simulink model "MavicProComplete"  (R2019a)
settings: Solver=VariableStepAuto  StartTime=0  StopTime=250  FixedStep=.01  MaxStep=10  MinStep=.001  RelTol=1e-4  EnableMultiTasking=on
InitFcn:
  | addpath params;
  | addpath fcns;
  | load batteryParams;
  | load motorParams;
  | load ukfBatteryParams;
  | load DJI.mat;
  | load DJIquadModel_X.mat;
model workspace (MAT data in the model file):
  Sig = Simulink.Signal
  Sig.DataType = 'auto'
  Sig.Dimensions = -1
  Sig.DimensionsMode = 'auto'
  Sig.Complexity = 'auto'
  Sig.SampleTime = -1
  Sig.SamplingMode = 'auto'
undefined symbols (not defined in the file): motorRes, P, Phi, Psi, Q, quadModel, R, The, Z
libraries: simulink x7, dspstat3 x5
(part 1 of 2)
Description:
  | This is a configurable quadcopter simulation.
  | This Simulink model demonstates attitude control.
  | 
  | Additional quadcopter modeling and simulation materials available at:
  | github.com/dch33/Quad-Sim
  | 
  | Copyright (C) 2014 D. Hartman, K. Landis, S. Moreno, J. Kim, M. Mehrer
  | 
  | License:
  |     This program is free software: you can redistribute it and/or modify
  |     it under the terms of the GNU LESSER GENERAL PUBLIC LICENSE as published by
  |     the Free Software Foundation, either version 3 of the License, or
  |     (at your option) any later version.
  | 
  |     This program is distributed in the hope that it will be useful,
  |     but WITHOUT ANY WARRANTY; without even the implied warranty of
  |     MERCHANTABILITY or FITNESS FOR A PARTICULAR PURPOSE.  See the
  |     GNU General Public License for more details.
  | 
  |     You should have received a copy of the GNU LESSER GENERAL PUBLIC LICENSE
  |     along with this program.  If not, see <http://www.gnu.org/licenses/>.
settings Model: ModifiedComment=tdarrah -- Tue Jun 04 09:34:35 2019 -- Version 1.40  Creator=David Hartman  LastModifiedBy=tdarrah
settings Model: ModifiedHistory=|
  | tdarrah -- Tue Jun 04 09:34:35 2019 -- Version 1.40
  | 
  | tdarrah -- Tue Jun 04 05:29:55 2019 -- Version 1.39
  | 
  | tdarrah -- Mon Jun 03 18:31:35 2019 -- Version 1.38
  | closed the battery loop
  | 
  | tdarrah -- Mon Jun 03 18:20:30 2019 -- Version 1.37
  | added battery
  | 
  | 
  | tdarrah -- Mon Jun 03 17:58:08 2019 -- Version 1.36
  | incorporated our motors in model
  | 
  | 
  | Sahai Couso -- Fri May 10 11:35:12 2019 -- Version 1.35
  | 
  | Sahai Couso -- Fri May 10 10:41:34 2019 -- Version 1.34
  | 
  | Sahai Couso -- Fri May 10 10:40:52 2019 -- Version 1.33
  | 
  | Sahai Couso -- Fri May 10 10:30:50 2019 -- Version 1.32
  | 
  | Sahai Couso -- Fri May 10 10:24:25 2019 -- Version 1.31
  | 
  | Sahai Couso -- Wed May 08 22:16:35 2019 -- Version 1.30
  | 
  | Sahai Couso -- Wed May 08 22:15:23 2019 -- Version 1.29
  | 
  | Sahai Couso -- Wed May 08 22:14:58 2019 -- Version 1.28
  | 
  | Sahai Couso -- Wed May 08 22:04:36 2019 -- Version 1.27
  | 
  | Sahai Couso -- Wed May 08 22:04:16 2019 -- Version 1.26
  | 
  | Sahai Couso -- Wed May 08 21:57:14 2019 -- Version 1.25
  | 
  | Sahai Couso -- Wed May 08 21:54:04 2019 -- Version 1.24
  | 
  | Sahai Couso -- Wed May 08 21:53:17 2019 -- Version 1.23
  | 
  | Sahai Couso -- Wed May 08 21:48:07 2019 -- Version 1.22
  | 
  | Sahai Couso -- Wed May 08 21:35:53 2019 -- Version 1.21
  | 
  | Sahai Couso -- Wed May 08 21:28:21 2019 -- Version 1.19
  | 
  | Sahai Couso -- Wed May 08 21:28:21 2019 -- Version 1.19
  | 
  | Sahai Couso -- Wed May 08 21:25:30 2019 -- Version 1.18
  | 
  | Sahai Couso -- Wed May 08 21:23:06 2019 -- Version 1.17
  | 
  | Sahai Couso -- Wed May 08 13:57:34 2019 -- Version 1.16
  | 
  | Sahai Couso -- Wed May 08 00:58:43 2019 -- Version 1.15
  | 
  | Sahai Couso -- Wed May 08 00:58:03 2019 -- Version 1.14
  | 
  | Sahai Couso -- Tue May 07 23:55:58 2019 -- Version 1.13
  | 
  | Sahai Couso -- Tue May 07 23:08:00 2019 -- Version 1.12
  | 
  | Sahai Couso -- Tue May 07 23:06:52 2019 -- Version 1.11
  | 
  | Sahai Couso -- Tue May 07 22:57:09 2019 -- Version 1.10
  | 
  | Sahai Couso -- Tue May 07 22:48:57 2019 -- Version 1.9
  | 
  | Sahai Couso -- Tue May 07 21:40:08 2019 -- Version 1.8
  | 
  | Yves -- Tue Apr 04 13:12:37 2017 -- Version 1.7
  | 
  | Yves -- Tue Apr 04 13:10:33 2017 -- Version 1.6
  | 
  | davidhartman -- Fri Jun 06 23:19:51 2014 -- Version 1.5
  | 
  | 
  | davidhartman -- Fri Jun 06 22:53:10 2014 -- Version 1.3
settings SolverCC: AlgebraicLoopSolver=LineSearch  AutoInsertRateTranBlk=on
settings DataIOCC: SaveFormat=Array  SignalLogging=off  ReturnWorkspaceOutputs=off
settings OptimizationCC: DefaultParameterBehavior=Inlined  LifeSpan=inf
settings DebuggingCC: UnderspecifiedInitializationDetection=Classic  MergeDetectMultiDrivingBlocksExec=none  SolverPrmCheckMsg=warning  UniqueDataStoreMsg=warning  StateNameClashWarn=warning  StrictBusMsg=WarnOnBusTreatedAsVector  SFUnexpectedBacktrackingDiag=warning  SFNoUnconditionalDefaultTransitionDiag=warning  SFExecutionAtInitializationDiag=none  ArithmeticOperatorsInVariantConditions=warning
settings HardwareCC: ProdBitPerPointer=32  ProdBitPerSizeT=32  ProdBitPerPtrDiffT=32  ProdLargestAtomicFloat=None  ProdIntDivRoundTo=Undefined  ProdEndianess=Unspecified  ProdWordSize=32  ProdHWDeviceType=32-bit Generic
settings ModelReferenceCC: PropagateSignalLabelsOutOfModel=off
settings SFSimCC: SimUseLocalCustomCode=off
settings RTWCC: RTWUseLocalCustomCode=off
settings CodeAppCC: StateflowObjectComments=on
settings GRTTargetCC: TargetLangStandard=C89/C90 (ANSI)  GeneratePreprocessorConditionals=Disable all
settings ConfigComp: CovMetricSettings=dw  CovHtmlReporting=on  CovSaveCumulativeToWorkspaceVar=on  CovSaveSingleToWorkspaceVar=on  CovExternalEMLEnable=off

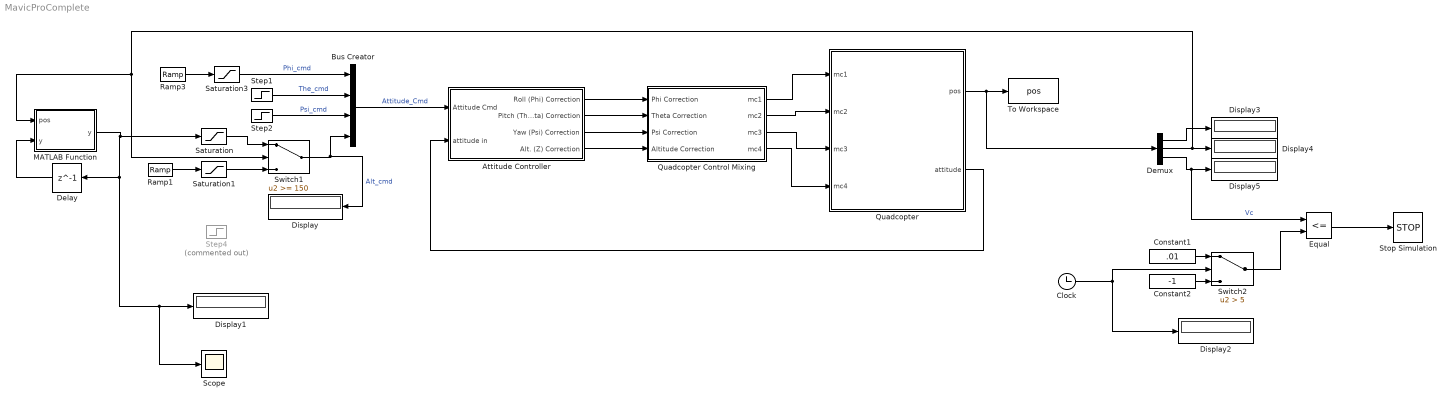
== system MavicProComplete ==
  Attitude Controller : Subsystem
  Bus Creator : BusCreator  Inputs=4
  Clock : Clock
  Constant1 : Constant  Value=.01
  Constant2 : Constant  Value=-1
  Delay : Delay  DelayLength=1  InitialCondition=10
  Demux : Demux  Outputs=3
  Display{,1..5} (6 alike) : Display
  Equal : RelationalOperator  Operator=<=  OutDataTypeStr=boolean  RndMeth=Simplest
  MATLAB Function : MATLAB Function  TreatAsAtomicUnit=on  SystemSampleTime=.1
      settings: MinAlgLoopOccurrences=on
  Quadcopter : Subsystem
  Quadcopter Control Mixing : Subsystem
  Ramp1 : simulink/Sources/Ramp  slope=.1  start=0  InitialOutput=0
  Ramp3 : simulink/Sources/Ramp  slope=-.0001  start=0  InitialOutput=0
  Saturation : Saturate  UpperLimit=10  LowerLimit=-1
  Saturation1 : Saturate  UpperLimit=10  LowerLimit=0
  Saturation3 : Saturate  UpperLimit=.002  LowerLimit=-.002
  Scope : Scope
  Step1 : Step  Time=1000000  After=10*pi/180  SampleTime=1
  Step2 : Step  Time=1000000  After=45*pi/180  SampleTime=1
  Step4 : Step  Commented=on  Time=0  Before=10  After=10  SampleTime=0
  Stop Simulation : Stop
  Switch1 : Switch  Threshold=150
  Switch2 : Switch  Criteria=u2 > Threshold  Threshold=5
  To Workspace : ToWorkspace  VariableName=pos  SampleTime=-1
      settings: Save2DSignal=2-D array (concatenate along first dimension)
  wires:
  Quadcopter/2(attitude) -> Attitude Controller/2(attitude in)
  Quadcopter Control Mixing/1(mc1) -> Quadcopter/1(mc1)
  Quadcopter Control Mixing/2(mc2) -> Quadcopter/2(mc2)
  Quadcopter Control Mixing/3(mc3) -> Quadcopter/3(mc3)
  Quadcopter Control Mixing/4(mc4) -> Quadcopter/4(mc4)
  Attitude Controller/1(Roll (Phi) Correction) -> Quadcopter Control Mixing/1(Phi Correction)
  Attitude Controller/2(Pitch (Theta) Correction) -> Quadcopter Control Mixing/2(Theta Correction)
  Attitude Controller/3(Yaw (Psi) Correction) -> Quadcopter Control Mixing/3(Psi Correction)
  Attitude Controller/4(Alt. (Z) Correction) -> Quadcopter Control Mixing/4(Altitude Correction)
  Saturation/1 -> Switch1/1
  Saturation3/1 -> Bus Creator/1  "Phi_cmd"
  Bus Creator/1 -> Attitude Controller/1(Attitude Cmd)  "Attitude_Cmd"
  Step2/1 -> Bus Creator/3  "Psi_cmd"
  Step1/1 -> Bus Creator/2  "The_cmd"
  Quadcopter/1(pos) -> Demux/1, To Workspace/1
  Saturation1/1 -> Switch1/3
  Ramp1/1 -> Saturation1/1
  Switch1/1 -> Display/1, Bus Creator/4  "Alt_cmd"
  Ramp3/1 -> Saturation3/1
  Demux/1 -> Display3/1
  Demux/2 -> MATLAB Function/1(pos), Switch1/2, Display4/1
  Demux/3 -> Equal/1, Display5/1  "Vc"
  Equal/1 -> Stop Simulation/1
  Constant1/1 -> Switch2/1
  Constant2/1 -> Switch2/3
  Switch2/1 -> Equal/2
  Clock/1 -> Switch2/2, Display2/1
  MATLAB Function/1(y) -> Scope/1, Display1/1, Delay/1, Saturation/1
  Delay/1 -> MATLAB Function/2("y ")

== system MavicProComplete/Attitude Controller ==
  Attitude Cmd : Inport
  attitude in : Inport  Port=2
  Altitude (Z) Control : Subsystem  mask{Kpz=3.0, Kiz=4.5, Kdz=3.0, LimitOutput=on, USat=1, LSat=-1, GOffset=(sqrt((quadModel.mass*quadModel.g)/(4*quadModel.ct))-quadModel.b)/quadModel.cr}
      mask prompts: Kpz "Kp"; Kiz "Ki"; Kdz "Kd"; LimitOutput "Integral Saturation?"; USat "Upper saturation limit:"; LSat "Lower saturation limit:"; GOffset "Gravity Feedforward"
      mask help:
      | Adjust PID controller gains through this mask interface, or "look under mask" for more detailed adjustments.
      |
      | Note: Gravity Offset will not appear on block face as a value until simulation is run if it is the result of a formula involving the quadcopter model parameters.
      mask TypeOptions Kpz: Kpz/Gain
      mask TypeOptions Kiz: Kiz/Gain
      mask TypeOptions Kdz: Kdz/Gain
      mask TypeOptions LimitOutput:
      | Integrator
      | Limited/LimitOutput
      mask TypeOptions USat:
      | Integrator
      | Limited/UpperSaturationLimit
      mask TypeOptions LSat:
      | Integrator
      | Limited/LowerSaturationLimit
      mask TypeOptions GOffset: Gravity Offset (Level Flight)/Value
      mask Display:
      | fprintf(['Gravity Offset = ' num2str(GOffset) '\n' ...
      |     'Kp = ' num2str(Kpz) '\n' ...
      |     'Ki = ' num2str(Kiz) '\n' ...
      |     'Kd = ' num2str(Kdz) '\n' ...
      |     'Integral Saturation: ' LimitOutput]);
      | if strcmp(LimitOutput,'on')
      |     fprintf([' \n' ' \n' ' \n' ' \n' ' \n' '\n' ...
      |         'Limits: ' num2str(USat) ' to ' num2str(LSat)]);
      | end
  Bus Selector : BusSelector  OutputSignals=Phi,P,The,Q,Psi,R,Z
  Pitch (Theta) Control : Subsystem  mask{Kpt=2, Kit=1.1, Kdt=1.2, LimitOutput=on, USat=1, LSat=-1}
      mask prompts: Kpt "Kp"; Kit "Ki"; Kdt "Kd"; LimitOutput "Integral Saturation?"; USat "Upper saturation limit:"; LSat "Lower saturation limit:"
      mask help: Adjust PID controller gains through this mask interface, or "look under mask" for more detailed adjustments.
      mask TypeOptions Kpt: Kpt/Gain
      mask TypeOptions Kit: Kit/Gain
      mask TypeOptions Kdt: Kdt/Gain
      mask TypeOptions LimitOutput:
      | Integrator
      | Limited/LimitOutput
      mask TypeOptions USat:
      | Integrator
      | Limited/UpperSaturationLimit
      mask TypeOptions LSat:
      | Integrator
      | Limited/LowerSaturationLimit
      mask Display:
      | fprintf(['Kp = ' num2str(Kpt) '\n' ...
      |     'Ki = ' num2str(Kit) '\n' ...
      |     'Kd = ' num2str(Kdt) '\n' ...
      |     'Integral Saturation: ' LimitOutput]);
      | if strcmp(LimitOutput,'on')
      |     fprintf([' \n' ' \n' ' \n' ' \n' '\n' ...
      |         'Limits: ' num2str(USat) ' to ' num2str(LSat)]);
      | end
  "Roll (Phi) Control " : Subsystem  mask{Kpp=2.0, Kip=1.1, Kdp=1.2, LimitOutput=on, USat=1, LSat=-1}
      mask prompts: Kpp "Kp"; Kip "Ki"; Kdp "Kd"; LimitOutput "Integral Saturation:"; USat "Upper saturation limit:"; LSat "Lower saturation limit:"
      mask help:
      | Adjust PID controller gains through this mask interface, or "look under mask"
      | for more detailed adjustments.
      mask TypeOptions Kpp: Kpp/Gain
      mask TypeOptions Kip: Kip/Gain
      mask TypeOptions Kdp: Kdp/Gain
      mask TypeOptions LimitOutput:
      | Integrator
      | Limited/LimitOutput
      mask TypeOptions USat:
      | Integrator
      | Limited/UpperSaturationLimit
      mask TypeOptions LSat:
      | Integrator
      | Limited/LowerSaturationLimit
      mask Display:
      | fprintf(['Kp = ' num2str(Kpp) '\n' ...
      |     'Ki = ' num2str(Kip) '\n' ...
      |     'Kd = ' num2str(Kdp) '\n'...
      |     'Integral Saturation: ' LimitOutput]);
      | if strcmp(LimitOutput,'on')
      |     fprintf([' \n' ' \n' ' \n' ' \n' '\n' ...
      |         'Limits: ' num2str(USat) ' to ' num2str(LSat)]);
      | end
  Yaw (Psi) Control : Subsystem  mask{Kps=4, Kis=0.5, Kds=3.5, LimitOutput=on, USat=1, LSat=-1}
      mask prompts: Kps "Kp"; Kis "Ki"; Kds "Kd"; LimitOutput "Integral Saturation?"; USat "Upper saturation limit:"; LSat "Lower saturation limit:"
      mask help: Adjust PID controller gains through this mask interface, or "look under mask" for more detailed adjustments.
      mask TypeOptions Kps: Kps/Gain
      mask TypeOptions Kis: Kit/Gain
      mask TypeOptions Kds: Kds/Gain
      mask TypeOptions LimitOutput:
      | Integrator
      | Limited/LimitOutput
      mask TypeOptions USat:
      | Integrator
      | Limited/UpperSaturationLimit
      mask TypeOptions LSat:
      | Integrator
      | Limited/LowerSaturationLimit
      mask Display:
      | fprintf(['Kp = ' num2str(Kps) '\n' ...
      |     'Ki = ' num2str(Kis) '\n' ...
      |     'Kd = ' num2str(Kds) '\n' ...
      |     'Integral Saturation: ' LimitOutput]);
      | if strcmp(LimitOutput,'on')
      |     fprintf([' \n' ' \n' ' \n' ' \n' '\n' ...
      |         'Limits: ' num2str(USat) ' to ' num2str(LSat)]);
      | end
  Roll (Phi) Correction : Outport
  Pitch (Theta) Correction : Outport  Port=2
  Yaw (Psi) Correction : Outport  Port=3
  Alt. (Z) Correction : Outport  Port=4
  wires:
  Bus Selector/6 -> Yaw (Psi) Control/3(R State)  "<R>"
  Bus Selector/4 -> Pitch (Theta) Control/3(Q State)  "<Q>"
  Bus Selector/2 -> "Roll (Phi) Control "/3(P)  "<P>"
  Bus Selector/3 -> Pitch (Theta) Control/2(Theta State)  "<The>"
  Attitude Cmd/1 -> "Roll (Phi) Control "/1("Attitude Command "), Pitch (Theta) Control/1(Attitude Command), Yaw (Psi) Control/1(Attitude Command), Altitude (Z) Control/1(Desired Z)
  Bus Selector/7 -> Altitude (Z) Control/2(Z State)  "<Z>"
  Altitude (Z) Control/1(Alt. (Z) Correction) -> Alt. (Z) Correction/1
  Bus Selector/5 -> Yaw (Psi) Control/2(Psi State)  "<Psi>"
  Yaw (Psi) Control/1(Psi Correction) -> Yaw (Psi) Correction/1
  Pitch (Theta) Control/1(Theta Correction) -> Pitch (Theta) Correction/1
  attitude in/1 -> Bus Selector/1
  Bus Selector/1 -> "Roll (Phi) Control "/2(Phi State)  "<Phi>"
  "Roll (Phi) Control "/1(Phi Correction) -> Roll (Phi) Correction/1

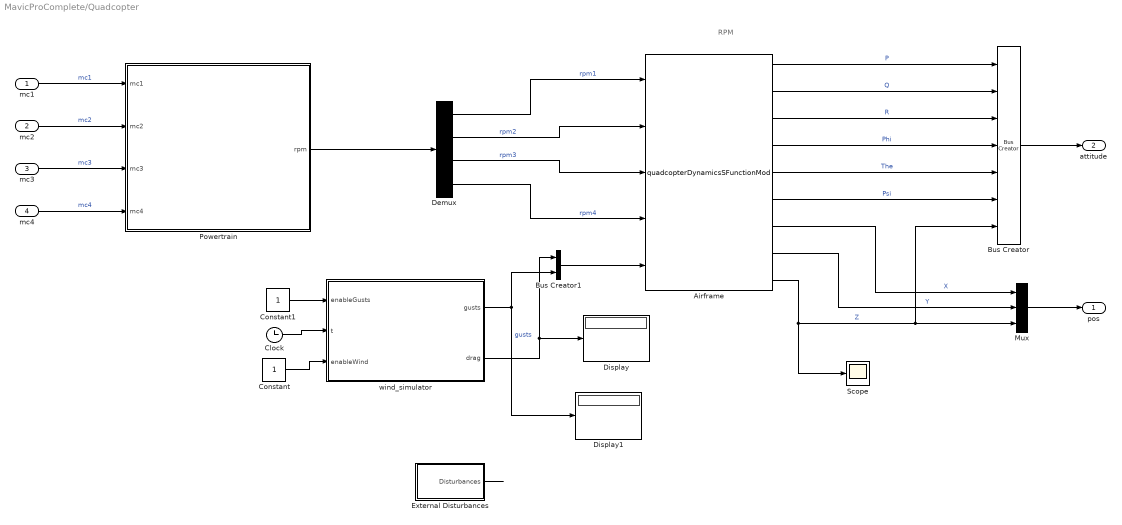
== system MavicProComplete/Quadcopter ==
  note: RPM
  mc1 : Inport
  mc2 : Inport  Port=2
  mc3 : Inport  Port=3
  mc4 : Inport  Port=4
  Airframe : M-S-Function  FunctionName=quadcopterDynamicsSFunctionMod  Parameters=quadModel, IC
      mask Display:
      | port_label('input', 1, 'RPM1')
      | port_label('input', 2, 'RPM2')
      | port_label('input', 3, 'RPM3')
      | port_label('input', 4, 'RPM4')
      | port_label('input', 5, 'Disturbances')
      | port_label('output', 1, 'P')
      | port_label('output', 2, 'Q')
      | port_label('output', 3, 'R')
      | port_label('output', 4, 'Phi')
      | port_label('output', 5, 'The')
      | port_label('output', 6, 'Psi')
      | port_label('output', 7, 'X')
      | port_label('output', 8, 'Y')
      | port_label('output', 9, 'Z')
  Bus Creator : BusCreator  Inputs=P,Q,R,Phi,The,Psi,Z
  Bus Creator1 : BusCreator  Inputs=2
  Clock : Clock
  Constant : Constant
  Constant1 : Constant
  Demux : Demux
  Display : Display
  Display1 : Display
  External Disturbances : Subsystem
  Mux : Mux  Inputs=3
  Powertrain : Subsystem
  Scope : Scope
  wind_simulator : Subsystem
  pos : Outport
  attitude : Outport  Port=2
  wires:
  External Disturbances/1("Disturbances ") -> ?
  Bus Creator/1 -> attitude/1
  Airframe/9 -> Scope/1, Bus Creator/7, Mux/3  "Z"
  Airframe/8 -> Mux/2  "Y"
  Airframe/7 -> Mux/1  "X"
  Airframe/6 -> Bus Creator/6  "Psi"
  Airframe/5 -> Bus Creator/5  "The"
  Airframe/4 -> Bus Creator/4  "Phi"
  Airframe/3 -> Bus Creator/3  "R"
  Airframe/2 -> Bus Creator/2  "Q"
  Airframe/1 -> Bus Creator/1  "P"
  Mux/1 -> pos/1
  Demux/1 -> Airframe/1  "rpm1"
  Demux/2 -> Airframe/2  "rpm2"
  Demux/3 -> Airframe/3  "rpm3"
  Demux/4 -> Airframe/4  "rpm4"
  mc1/1 -> Powertrain/1(mc1)  "mc1"
  mc2/1 -> Powertrain/2(mc2)  "mc2"
  mc3/1 -> Powertrain/3(mc3)  "mc3"
  mc4/1 -> Powertrain/4(mc4)  "mc4"
  Powertrain/1(rpm) -> Demux/1
  wind_simulator/2(drag) -> Bus Creator1/1, Display/1
  Constant/1 -> wind_simulator/3(enableWind)
  Constant1/1 -> wind_simulator/1(enableGusts)
  Clock/1 -> wind_simulator/2(t)
  wind_simulator/1(gusts) -> Bus Creator1/2, Display1/1  "gusts"
  Bus Creator1/1 -> Airframe/5

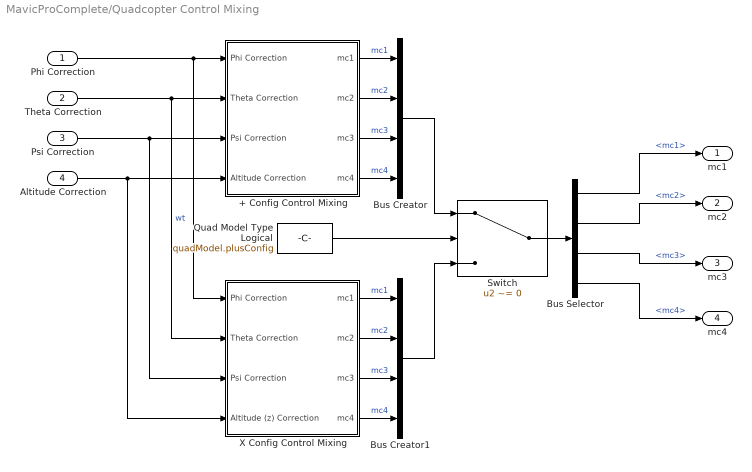
== system MavicProComplete/Quadcopter Control Mixing ==
  Phi Correction : Inport
  Theta Correction : Inport  Port=2
  Psi Correction : Inport  Port=3
  Altitude Correction : Inport  Port=4
  + Config Control Mixing : Subsystem
  Bus Creator : BusCreator  Inputs=4
  Bus Creator1 : BusCreator  Inputs=4
  Bus Selector : BusSelector  OutputSignals=mc1,mc2,mc3,mc4
  Quad Model Type Logical : Constant  Value=quadModel.plusConfig
  Switch : Switch  Criteria=u2 ~= 0
  X Config Control Mixing : Subsystem
  mc1 : Outport
  mc2 : Outport  Port=2
  mc3 : Outport  Port=3
  mc4 : Outport  Port=4
  wires:
  Switch/1 -> Bus Selector/1
  Quad Model Type Logical/1 -> Switch/2
  Bus Selector/4 -> mc4/1  "<mc4>"
  Bus Selector/3 -> mc3/1  "<mc3>"
  Bus Selector/2 -> mc2/1  "<mc2>"
  Bus Selector/1 -> mc1/1  "<mc1>"
  Bus Creator1/1 -> Switch/3
  X Config Control Mixing/4(mc4) -> Bus Creator1/4  "mc4"
  X Config Control Mixing/3(mc3) -> Bus Creator1/3  "mc3"
  X Config Control Mixing/2(mc2) -> Bus Creator1/2  "mc2"
  X Config Control Mixing/1(mc1) -> Bus Creator1/1  "mc1"
  Bus Creator/1 -> Switch/1
  + Config Control Mixing/4(mc4) -> Bus Creator/4  "mc4"
  + Config Control Mixing/3(mc3) -> Bus Creator/3  "mc3"
  + Config Control Mixing/2(mc2) -> Bus Creator/2  "mc2"
  + Config Control Mixing/1(mc1) -> Bus Creator/1  "mc1"
  Altitude Correction/1 -> + Config Control Mixing/4(Altitude Correction), X Config Control Mixing/4(Altitude (z) Correction)
  Psi Correction/1 -> + Config Control Mixing/3(Psi Correction), X Config Control Mixing/3(Psi Correction)
  Theta Correction/1 -> + Config Control Mixing/2(Theta Correction), X Config Control Mixing/2(Theta Correction)  "wt"
  Phi Correction/1 -> + Config Control Mixing/1(Phi Correction), X Config Control Mixing/1(Phi Correction)

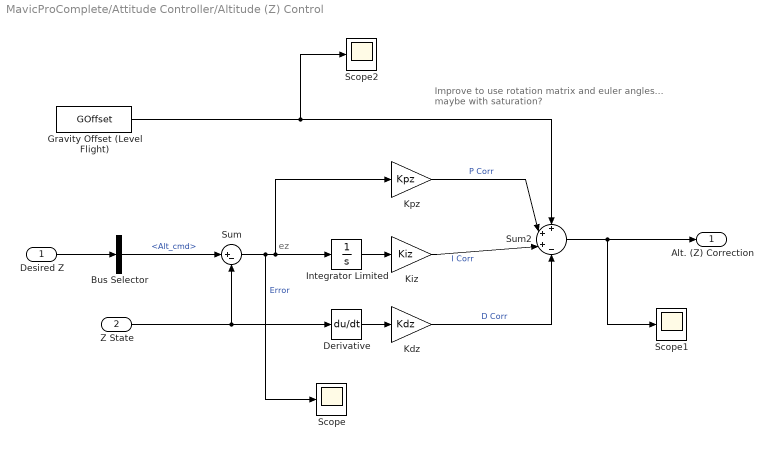
== system MavicProComplete/Attitude Controller/Altitude (Z) Control ==
  note: ez
  note: Improve to use rotation matrix and euler angles...
      | maybe with saturation?
  Desired Z : Inport
  Z State : Inport  Port=2
  Bus Selector : BusSelector  OutputSignals=Alt_cmd
  Derivative : Derivative
  Gravity Offset (Level Flight) : Constant  Value=GOffset
  Integrator Limited : Integrator  LimitOutput=on  UpperSaturationLimit=USat  LowerSaturationLimit=LSat
  Kdz : Gain  Gain=Kdz
  Kiz : Gain  Gain=Kiz
  Kpz : Gain  Gain=Kpz
  Scope : Scope
  Scope1 : Scope
  Scope2 : Scope
  Sum : Sum  Inputs=|+-
  Sum2 : Sum  Inputs=+++-
  Alt. (Z) Correction : Outport
  wires:
  Derivative/1 -> Kdz/1
  Bus Selector/1 -> Sum/1  "<Alt_cmd>"
  Integrator Limited/1 -> Kiz/1
  Kdz/1 -> Sum2/4  "D Corr"
  Kiz/1 -> Sum2/3  "I Corr"
  Sum/1 -> Scope/1, Kpz/1, Integrator Limited/1  "Error"
  Kpz/1 -> Sum2/2  "P Corr"
  Sum2/1 -> Scope1/1, Alt. (Z) Correction/1
  Z State/1 -> Sum/2, Derivative/1
  Desired Z/1 -> Bus Selector/1
  Gravity Offset (Level Flight)/1 -> Scope2/1, Sum2/1

== system MavicProComplete/Attitude Controller/Pitch (Theta) Control ==
  Attitude Command : Inport
  Theta State : Inport  Port=2
  Q State : Inport  Port=3
  Bus Selector : BusSelector  OutputSignals=The_cmd
  Integrator Limited : Integrator  LimitOutput=on  UpperSaturationLimit=USat  LowerSaturationLimit=LSat
  Kdt : Gain  Gain=Kdt
  Kit : Gain  Gain=Kit
  Kpt : Gain  Gain=Kpt
  Sum : Sum  Inputs=|+-
  Sum1 : Sum  Inputs=++-
  Theta Correction : Outport
  wires:
  Q State/1 -> Kdt/1
  Bus Selector/1 -> Sum/1  "<The_cmd>"
  Integrator Limited/1 -> Kit/1
  Kit/1 -> Sum1/2  "I Corr"
  Kdt/1 -> Sum1/3  "D Corr"
  Kpt/1 -> Sum1/1  "P Corr"
  Sum1/1 -> Theta Correction/1
  Theta State/1 -> Sum/2
  Attitude Command/1 -> Bus Selector/1
  Sum/1 -> Kpt/1, Integrator Limited/1  "Error"

== system MavicProComplete/Attitude Controller/Roll (Phi) Control  ==
  "Attitude Command " : Inport
  Phi State : Inport  Port=2
  P : Inport  Port=3
  Bus Selector : BusSelector  OutputSignals=Phi_cmd
  Integrator Limited : Integrator  LimitOutput=on  UpperSaturationLimit=USat  LowerSaturationLimit=LSat
  Kdp : Gain  Gain=Kdp
  Kip : Gain  Gain=Kip
  Kpp : Gain  Gain=Kpp
  Sum : Sum  Inputs=|+-
  Sum1 : Sum  Inputs=++-
  Phi Correction : Outport
  wires:
  P/1 -> Kdp/1
  Bus Selector/1 -> Sum/1  "<Phi_cmd>"
  "Attitude Command "/1 -> Bus Selector/1
  Integrator Limited/1 -> Kip/1
  Kip/1 -> Sum1/2  "I Corr"
  Kdp/1 -> Sum1/3  "D Corr"
  Kpp/1 -> Sum1/1  "P Corr"
  Sum1/1 -> Phi Correction/1
  Phi State/1 -> Sum/2
  Sum/1 -> Kpp/1, Integrator Limited/1  "Error"

== system MavicProComplete/Attitude Controller/Yaw (Psi) Control ==
  Attitude Command : Inport
  Psi State : Inport  Port=2
  R State : Inport  Port=3
  Bus Selector : BusSelector  OutputSignals=Psi_cmd
  Integrator Limited : Integrator  LimitOutput=on  UpperSaturationLimit=USat  LowerSaturationLimit=LSat
  Kds : Gain  Gain=Kds
  Kit : Gain  Gain=Kis
  Kps : Gain  Gain=Kps
  Sum : Sum  Inputs=|+-
  Sum1 : Sum  Inputs=++-
  Psi Correction : Outport
  wires:
  R State/1 -> Kds/1
  Bus Selector/1 -> Sum/1  "<Psi_cmd>"
  Integrator Limited/1 -> Kit/1
  Kit/1 -> Sum1/2  "I Corr"
  Kds/1 -> Sum1/3  "D Corr"
  Kps/1 -> Sum1/1  "P Corr"
  Psi State/1 -> Sum/2
  Sum1/1 -> Psi Correction/1
  Attitude Command/1 -> Bus Selector/1
  Sum/1 -> Kps/1, Integrator Limited/1  "Error"

== system MavicProComplete/Quadcopter/External Disturbances ==
  note: Note: Torques are in units of N*m, Forces in N
      | Torques are applied to the BODY coordinate system.
      | Forces are applied from the WORLD coordinate system!
      | This can be changed by adjusting the equations within the S-function.
  Bus Creator : BusCreator  Inputs=6
  Bus to Vector : BusToVector
  Constant{2..6} (5 alike) : Constant  Value=0
  Step : Step  After=0  SampleTime=0
  "Disturbances " : Outport
  wires:
  Constant5/1 -> Bus Creator/6  "Force_z-axis"
  Constant4/1 -> Bus Creator/5  "Force_y-axis"
  Constant3/1 -> Bus Creator/4  "Force_x-axis"
  Constant2/1 -> Bus Creator/3  "Tau_bz-axis"
  Step/1 -> Bus Creator/2  "Tau_by-axis"
  Constant6/1 -> Bus Creator/1  "Tau_bx-axis"
  Bus Creator/1 -> Bus to Vector/1
  Bus to Vector/1 -> "Disturbances "/1

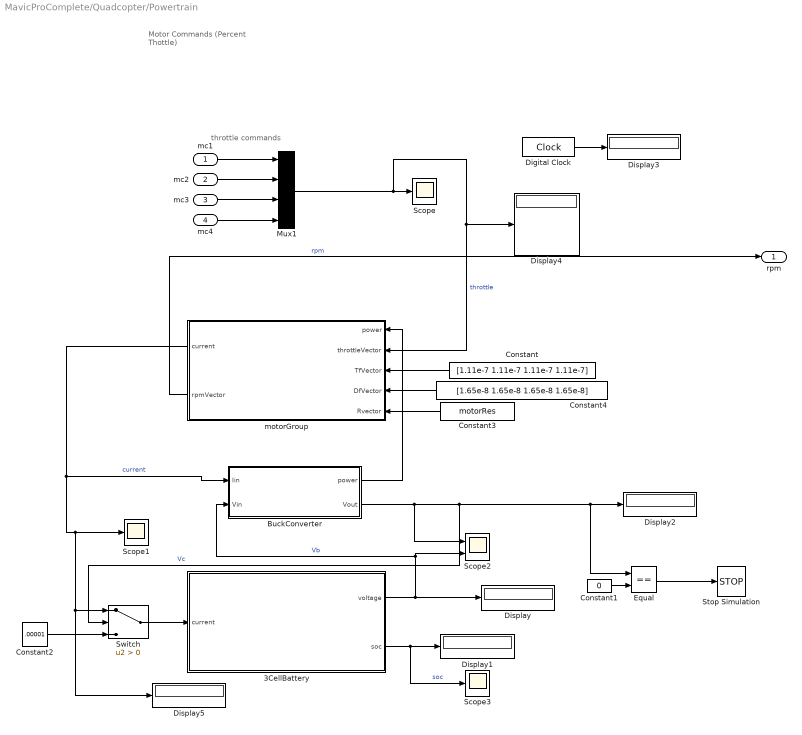
== system MavicProComplete/Quadcopter/Powertrain ==
  note: throttle commands
  note: Motor Commands
      | (Percent Thottle)
  mc1 : Inport
  mc2 : Inport  Port=2
  mc3 : Inport  Port=3
  mc4 : Inport  Port=4
  3CellBattery : Subsystem
  BuckConverter : Subsystem
  Constant : Constant  Value=[1.11e-7 1.11e-7 1.11e-7 1.11e-7]
  Constant1 : Constant  Value=0
  Constant2 : Constant  Value=.00001
  Constant3 : Constant  Value=motorRes
  Constant4 : Constant  Value=[1.65e-8 1.65e-8 1.65e-8 1.65e-8]
  Digital Clock : DigitalClock
      mask Display: disp('Sim Time');
  Display{,1..5} (6 alike) : Display
  Equal : RelationalOperator  Operator===  OutDataTypeStr=boolean  RndMeth=Simplest
  Mux1 : Mux
  Scope : Scope
  Scope1 : Scope
  Scope2 : Scope  NumInputPorts=2
  Scope3 : Scope
  Stop Simulation : Stop
  Switch : Switch  Criteria=u2 > Threshold
  motorGroup : Subsystem
  rpm : Outport
  wires:
  mc3/1 -> Mux1/3
  Digital Clock/1 -> Display3/1
  mc1/1 -> Mux1/1
  mc4/1 -> Mux1/4
  mc2/1 -> Mux1/2
  3CellBattery/1(voltage) -> Scope2/2, BuckConverter/2(Vin), Display/1  "Vb"
  motorGroup/2(rpmVector) -> rpm/1  "rpm"
  3CellBattery/2(soc) -> Display1/1, Scope3/1  "soc"
  Constant/1 -> motorGroup/3(TfVector)
  BuckConverter/2(Vout) -> Switch/2, Equal/1, Display2/1, Scope2/1  "Vc"
  BuckConverter/1(power) -> motorGroup/1(power)
  Constant1/1 -> Equal/2
  Constant4/1 -> motorGroup/4(DfVector)
  motorGroup/1(current) -> BuckConverter/1(Iin), Switch/1, Display5/1, Scope1/1  "current"
  Mux1/1 -> Display4/1, motorGroup/2(throttleVector), Scope/1  "throttle"
  Equal/1 -> Stop Simulation/1
  Switch/1 -> 3CellBattery/1(current)
  Constant2/1 -> Switch/3
  Constant3/1 -> motorGroup/5(Rvector)

== system MavicProComplete/Quadcopter/wind_simulator ==
  enableGusts : Inport
  t : Inport  Port=2
  enableWind : Inport  Port=3
  Constant10 : Constant  Value=.05
  Constant5 : Constant  Value=5
  Constant6 : Constant  Value=1.2
  Constant9 : Constant
  wind_and_gust : Subsystem
  gusts : Outport
  drag : Outport  Port=2
  wires:
  enableGusts/1 -> wind_and_gust/1(enableGusts)  "enableGusts"
  wind_and_gust/2(drag) -> drag/1  "drag"
  Constant6/1 -> wind_and_gust/3(amplitude)  "amplitude"
  Constant10/1 -> wind_and_gust/6(speed)  "speed"
  Constant9/1 -> wind_and_gust/5(windDirection)  "windDirection"
  wind_and_gust/1(gusts) -> gusts/1  "gusts"
  enableWind/1 -> wind_and_gust/7(enableWind)  "enableWind"
  t/1 -> wind_and_gust/4(t)
  Constant5/1 -> wind_and_gust/2(period)  "period"

== system MavicProComplete/Quadcopter Control Mixing/+ Config Control Mixing ==
  note: mc1 = Alt_cor -Psi_cor - The_cor
  note: mc3 = Alt_cor - Psi_cor + The_cor
  note: mc4 = Alt_cor + Psi_cor - Phi_cor
  note: + (plus) Quad Configuration Control Mixing
  note: mc2 = Alt_cor + Psi_cor + Phi_cor
  Phi Correction : Inport
  Theta Correction : Inport  Port=2
  Psi Correction : Inport  Port=3
  Altitude Correction : Inport  Port=4
  Sum1 : Sum  Inputs=|+-
  Sum11 : Sum  Inputs=-+|
  Sum2 : Sum  Inputs=|+-
  Sum3 : Sum  Inputs=++|
  Sum4 : Sum  Inputs=++|
  Sum8 : Sum  Inputs=|++
  mc1 : Outport
  mc2 : Outport  Port=2
  mc3 : Outport  Port=3
  mc4 : Outport  Port=4
  wires:
  Sum11/1 -> mc4/1
  Sum8/1 -> mc2/1
  Sum3/1 -> mc3/1
  Sum1/1 -> mc1/1
  Phi Correction/1 -> Sum11/1, Sum8/2
  Sum4/1 -> Sum8/1, Sum11/2
  Psi Correction/1 -> Sum2/2, Sum4/1
  Sum2/1 -> Sum1/1, Sum3/2
  Altitude Correction/1 -> Sum4/2, Sum2/1
  Theta Correction/1 -> Sum3/1, Sum1/2

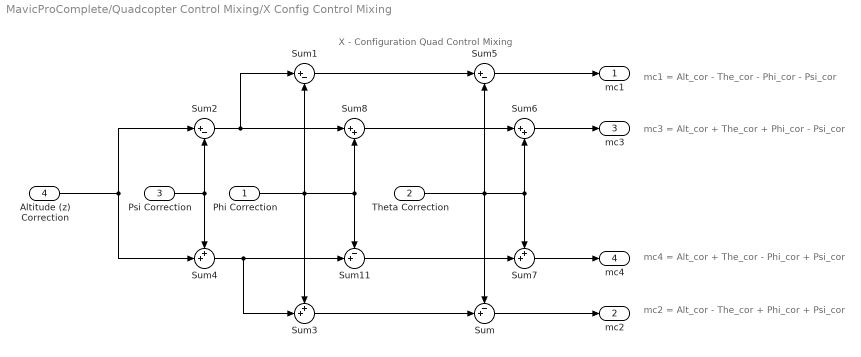
== system MavicProComplete/Quadcopter Control Mixing/X Config Control Mixing ==
  note: mc4 = Alt_cor + The_cor - Phi_cor + Psi_cor
  note: mc2 = Alt_cor - The_cor + Phi_cor + Psi_cor
  note: mc3 = Alt_cor + The_cor + Phi_cor - Psi_cor
  note: X - Configuration Quad Control Mixing
  note: mc1 = Alt_cor - The_cor - Phi_cor - Psi_cor
  Phi Correction : Inport
  Theta Correction : Inport  Port=2
  Psi Correction : Inport  Port=3
  Altitude (z) Correction : Inport  Port=4
  Sum : Sum  Inputs=-+|
  Sum1 : Sum  Inputs=|+-
  Sum11 : Sum  Inputs=-+|
  Sum2 : Sum  Inputs=|+-
  Sum3 : Sum  Inputs=++|
  Sum4 : Sum  Inputs=++|
  Sum5 : Sum  Inputs=|+-
  Sum6 : Sum  Inputs=|++
  Sum7 : Sum  Inputs=++|
  Sum8 : Sum  Inputs=|++
  mc1 : Outport
  mc2 : Outport  Port=2
  mc3 : Outport  Port=3
  mc4 : Outport  Port=4
  wires:
  Sum/1 -> mc2/1
  Altitude (z) Correction/1 -> Sum4/2, Sum2/1
  Sum7/1 -> mc4/1
  Sum6/1 -> mc3/1
  Sum5/1 -> mc1/1
  Sum11/1 -> Sum7/2
  Sum8/1 -> Sum6/1
  Sum1/1 -> Sum5/1
  Theta Correction/1 -> Sum/1, Sum5/2, Sum6/2, Sum7/1
  Sum3/1 -> Sum/2
  Sum4/1 -> Sum11/2, Sum3/2
  Phi Correction/1 -> Sum11/1, Sum8/2, Sum1/2, Sum3/1
  Psi Correction/1 -> Sum2/2, Sum4/1
  Sum2/1 -> Sum1/1, Sum8/1

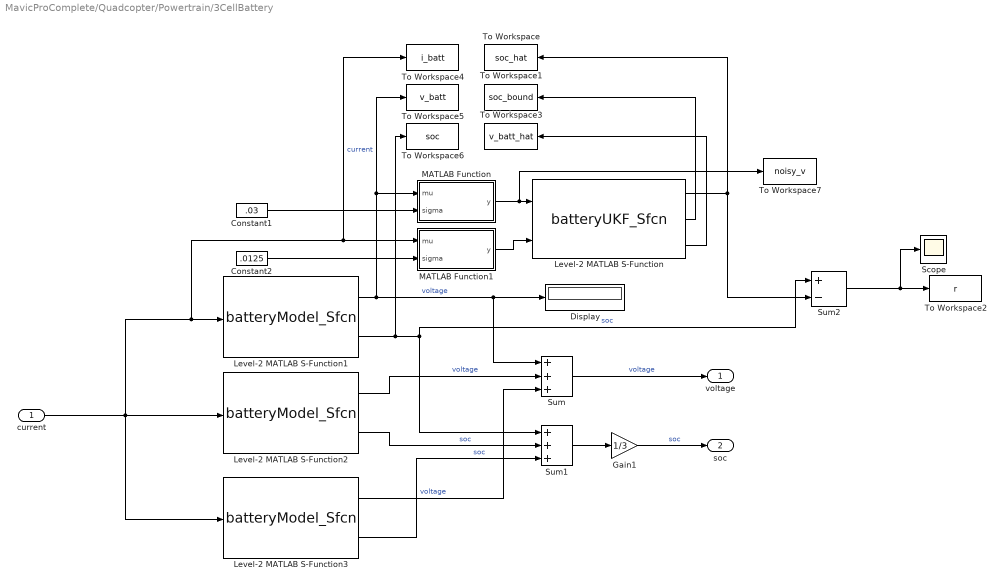
== system MavicProComplete/Quadcopter/Powertrain/3CellBattery ==
  current : Inport
  Constant1 : Constant  Value=.03
  Constant2 : Constant  Value=.0125
  Display : Display
  Gain1 : Gain  Gain=1/3
  Level-2 MATLAB S-Function : M-S-Function  FunctionName=batteryUKF_Sfcn  Parameters=batteryParams, batteryParams.dt, ukfBatteryParams
      mask Display:
      | port_label('input', 1, 'voltage');
      | port_label('input', 2, 'current');
      | port_label('output', 1, 'soc_hat');
      | port_label('output', 2, 'soc_bound');
      | port_label('output', 3, 'voltage_hat');
      | 
      | disp("UKF");
  Level-2 MATLAB S-Function1 : M-S-Function  FunctionName=batteryModel_Sfcn  Parameters=batteryParams, batteryParams.dt
      mask Display:
      | port_label('input', 1, 'current');
      | port_label('output', 1, 'voltage');
      | port_label('output', 2, 'soc');
      | 
      | disp("Battery Cell");
  Level-2 MATLAB S-Function2 : M-S-Function  FunctionName=batteryModel_Sfcn  Parameters=batteryParams, batteryParams.dt
      mask Display:
      | port_label('input', 1, 'current');
      | port_label('output', 1, 'voltage');
      | port_label('output', 2, 'soc');
      | 
      | disp("Battery Cell");
  Level-2 MATLAB S-Function3 : M-S-Function  FunctionName=batteryModel_Sfcn  Parameters=batteryParams, batteryParams.dt
      mask Display:
      | port_label('input', 1, 'current');
      | port_label('output', 1, 'voltage');
      | port_label('output', 2, 'soc');
      | 
      | disp("Battery Cell");
  MATLAB Function : MATLAB Function  TreatAsAtomicUnit=on
  MATLAB Function1 : MATLAB Function  TreatAsAtomicUnit=on
  Scope : Scope
  Sum : Sum  Inputs=+++
  Sum1 : Sum  Inputs=+++
  Sum2 : Sum  Inputs=+-
  To Workspace : ToWorkspace  VariableName=soc_hat  SaveFormat=Timeseries  SampleTime=-1
  To Workspace1 : ToWorkspace  VariableName=soc_bound  SaveFormat=Timeseries  SampleTime=-1
  To Workspace2 : ToWorkspace  VariableName=r  SaveFormat=Timeseries  SampleTime=-1
  To Workspace3 : ToWorkspace  VariableName=v_batt_hat  SaveFormat=Timeseries  SampleTime=-1
  To Workspace4 : ToWorkspace  VariableName=i_batt  SaveFormat=Timeseries  SampleTime=-1
  To Workspace5 : ToWorkspace  VariableName=v_batt  SaveFormat=Timeseries  SampleTime=-1
  To Workspace6 : ToWorkspace  VariableName=soc  SaveFormat=Timeseries  SampleTime=-1
  To Workspace7 : ToWorkspace  VariableName=noisy_v  SaveFormat=Timeseries  SampleTime=-1
  voltage : Outport
  soc : Outport  Port=2
  wires:
  Level-2 MATLAB S-Function2/1 -> Sum/2  "voltage"
  Level-2 MATLAB S-Function1/1 -> Display/1, Sum/1, MATLAB Function/1(mu), To Workspace5/1  "voltage"
  Level-2 MATLAB S-Function2/2 -> Sum1/2  "soc"
  Sum1/1 -> Gain1/1
  Gain1/1 -> soc/1  "soc"
  Level-2 MATLAB S-Function1/2 -> To Workspace6/1, Sum2/1, Sum1/1  "soc"
  Level-2 MATLAB S-Function3/2 -> Sum1/3  "soc"
  current/1 -> Level-2 MATLAB S-Function3/1, Level-2 MATLAB S-Function2/1, MATLAB Function1/1(mu), To Workspace4/1, Level-2 MATLAB S-Function1/1  "current"
  Level-2 MATLAB S-Function3/1 -> Sum/3  "voltage"
  Sum/1 -> voltage/1  "voltage"
  Level-2 MATLAB S-Function/1 -> Sum2/2, To Workspace/1
  Level-2 MATLAB S-Function/2 -> To Workspace1/1
  Sum2/1 -> Scope/1, To Workspace2/1
  Level-2 MATLAB S-Function/3 -> To Workspace3/1
  Constant1/1 -> MATLAB Function/2(sigma)
  MATLAB Function/1(y) -> To Workspace7/1, Level-2 MATLAB S-Function/1
  MATLAB Function1/1(y) -> Level-2 MATLAB S-Function/2
  Constant2/1 -> MATLAB Function1/2(sigma)

== system MavicProComplete/Quadcopter/Powertrain/BuckConverter ==
  Iin : Inport
  Vin : Inport  Port=2
  Constant : Constant  Value=0
  Constant2 : Constant  Value=11.4
  Product : Product
  Switch : Switch  Threshold=11.3
  power : Outport
  Vout : Outport  Port=2
  wires:
  Product/1 -> power/1
  Iin/1 -> Product/1
  Constant2/1 -> Switch/1
  Constant/1 -> Switch/3
  Vin/1 -> Switch/2
  Switch/1 -> Product/2, Vout/1

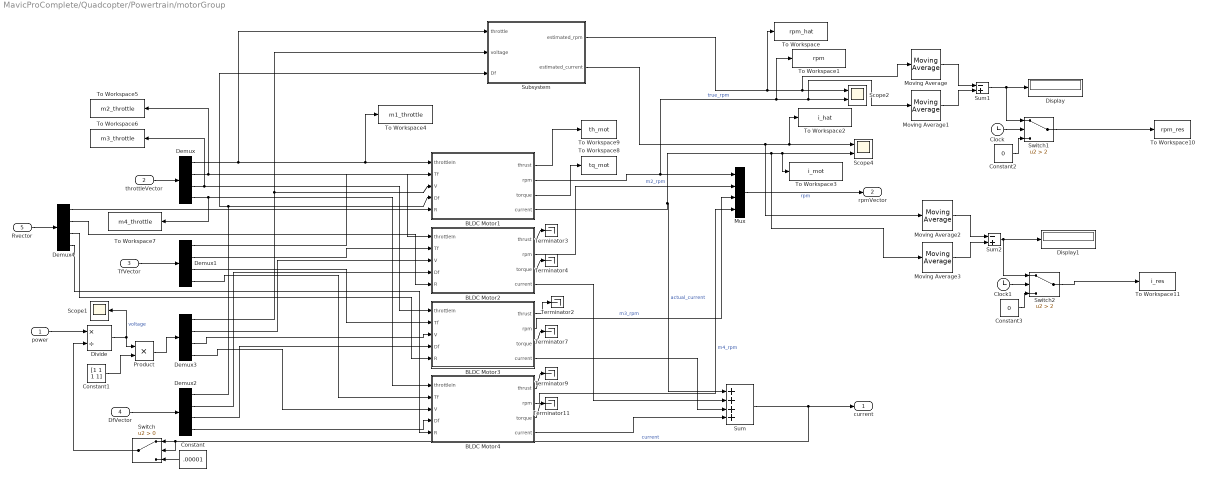
== system MavicProComplete/Quadcopter/Powertrain/motorGroup ==
  power : Inport
  throttleVector : Inport  Port=2  PortDimensions=4
  TfVector : Inport  Port=3  PortDimensions=4
  DfVector : Inport  Port=4
  Rvector : Inport  Port=5
  BLDC Motor1 : Subsystem
  BLDC Motor2 : Subsystem
  BLDC Motor3 : Subsystem
  BLDC Motor4 : Subsystem
  Clock : Clock
  Clock1 : Clock
  Constant : Constant  Value=.00001
  Constant1 : Constant  Value=[1 1 1 1]
  Constant2 : Constant  Value=0
  Constant3 : Constant  Value=0
  Demux{,1..4} (5 alike) : Demux
  Display : Display
  Display1 : Display
  Divide : Product  Inputs=*/
  Moving Average : dspstat3/Moving Average  Method=Sliding window  ForgettingFactorPort=off  SpecifyWindowLength=on  WindowLength=50  ForgettingFactor=0.9  SimulateUsing=Code generation
  Moving Average1 : dspstat3/Moving Average  Method=Sliding window  ForgettingFactorPort=off  SpecifyWindowLength=on  WindowLength=50  ForgettingFactor=0.9  SimulateUsing=Code generation
  Moving Average2 : dspstat3/Moving Average  Method=Sliding window  ForgettingFactorPort=off  SpecifyWindowLength=on  WindowLength=100  ForgettingFactor=0.9  SimulateUsing=Code generation
  Moving Average3 : dspstat3/Moving Average  Method=Sliding window  ForgettingFactorPort=off  SpecifyWindowLength=on  WindowLength=100  ForgettingFactor=0.9  SimulateUsing=Code generation
  Mux : Mux
  Product : Product
  Scope1 : Scope
  Scope2 : Scope  NumInputPorts=2
  Scope4 : Scope  NumInputPorts=2
  Subsystem : Subsystem
  Sum : Sum  Inputs=++++
  Sum1 : Sum  Inputs=-+
  Sum2 : Sum  Inputs=-+
  Switch : Switch  Criteria=u2 > Threshold
  Switch1 : Switch  Criteria=u2 > Threshold  Threshold=2
  Switch2 : Switch  Criteria=u2 > Threshold  Threshold=2
  Terminator{2..4,7,9,11} (6 alike) : Terminator
  To Workspace : ToWorkspace  VariableName=rpm_hat  SaveFormat=Timeseries  SampleTime=-1
  To Workspace1 : ToWorkspace  VariableName=rpm  SaveFormat=Timeseries  SampleTime=-1
  To Workspace10 : ToWorkspace  VariableName=rpm_res  SaveFormat=Timeseries  SampleTime=-1
  To Workspace11 : ToWorkspace  VariableName=i_res  SaveFormat=Timeseries  SampleTime=-1
  To Workspace2 : ToWorkspace  VariableName=i_hat  SaveFormat=Timeseries  SampleTime=-1
  To Workspace3 : ToWorkspace  VariableName=i_mot  SaveFormat=Timeseries  SampleTime=-1
  To Workspace4 : ToWorkspace  VariableName=m1_throttle  SaveFormat=Timeseries  SampleTime=-1
  To Workspace5 : ToWorkspace  VariableName=m2_throttle  SaveFormat=Timeseries  SampleTime=-1
  To Workspace6 : ToWorkspace  VariableName=m3_throttle  SaveFormat=Timeseries  SampleTime=-1
  To Workspace7 : ToWorkspace  VariableName=m4_throttle  SaveFormat=Timeseries  SampleTime=-1
  To Workspace8 : ToWorkspace  VariableName=tq_mot  SaveFormat=Timeseries  SampleTime=-1
  To Workspace9 : ToWorkspace  VariableName=th_mot  SaveFormat=Timeseries  SampleTime=-1
  current : Outport
  rpmVector : Outport  Port=2
  wires:
  Demux1/2 -> BLDC Motor2/2(Tf)
  Demux1/4 -> BLDC Motor4/2(Tf)
  Divide/1 -> Scope1/1, Product/1  "voltage"
  Demux1/1 -> BLDC Motor1/2(Tf)
  Sum/1 -> Switch/2, Switch/1, current/1  "current"
  Demux1/3 -> BLDC Motor3/2(Tf)
  BLDC Motor1/4(current) -> Moving Average3/1, To Workspace3/1, Scope4/2, Sum/1  "actual_current"
  power/1 -> Divide/1
  Demux/4 -> To Workspace7/1, BLDC Motor4/1(throttleIn)
  Demux/3 -> To Workspace6/1, BLDC Motor3/1(throttleIn)
  Demux/2 -> To Workspace5/1, BLDC Motor2/1(throttleIn)
  throttleVector/1 -> Demux/1
  TfVector/1 -> Demux1/1
  BLDC Motor4/4(current) -> Sum/4
  BLDC Motor3/4(current) -> Sum/3
  BLDC Motor2/4(current) -> Sum/2
  BLDC Motor4/2(rpm) -> Mux/4  "m4_rpm"
  BLDC Motor3/2(rpm) -> Mux/3  "m3_rpm"
  BLDC Motor2/2(rpm) -> Mux/2  "m2_rpm"
  BLDC Motor1/2(rpm) -> To Workspace1/1, Moving Average1/1, Scope2/2, Mux/1  "true_rpm"
  Mux/1 -> rpmVector/1  "rpm"
  BLDC Motor1/1(thrust) -> To Workspace9/1
  BLDC Motor4/3(torque) -> Terminator11/1
  BLDC Motor1/3(torque) -> To Workspace8/1
  BLDC Motor2/3(torque) -> Terminator4/1
  BLDC Motor3/3(torque) -> Terminator7/1
  BLDC Motor4/1(thrust) -> Terminator9/1
  BLDC Motor3/1(thrust) -> Terminator2/1
  BLDC Motor2/1(thrust) -> Terminator3/1
  Switch/1 -> Divide/2
  Constant/1 -> Switch/3
  Demux/1 -> Subsystem/1(throttle), To Workspace4/1, BLDC Motor1/1(throttleIn)
  Subsystem/1(estimated_rpm) -> To Workspace/1, Moving Average/1, Scope2/1
  DfVector/1 -> Demux2/1
  Demux2/1 -> BLDC Motor1/4(Df), Subsystem/3(Df)
  Demux2/2 -> BLDC Motor2/4(Df)
  Demux2/3 -> BLDC Motor3/4(Df)
  Demux2/4 -> BLDC Motor4/4(Df)
  Demux3/1 -> Subsystem/2(voltage), BLDC Motor1/3(V)
  Demux3/2 -> BLDC Motor2/3(V)
  Demux3/3 -> BLDC Motor3/3(V)
  Demux3/4 -> BLDC Motor4/3(V)
  Constant1/1 -> Product/2
  Product/1 -> Demux3/1
  Rvector/1 -> Demux4/1
  Demux4/1 -> BLDC Motor1/5(R)
  Demux4/2 -> BLDC Motor2/5(R)
  Demux4/3 -> BLDC Motor3/5(R)
  Demux4/4 -> BLDC Motor4/5(R)
  Moving Average1/1 -> Sum1/2
  Moving Average/1 -> Sum1/1
  Subsystem/2(estimated_current) -> Moving Average2/1, To Workspace2/1, Scope4/1
  Moving Average2/1 -> Sum2/1
  Moving Average3/1 -> Sum2/2
  Sum1/1 -> Switch1/1, Display/1
  Switch1/1 -> To Workspace10/1
  Constant2/1 -> Switch1/3
  Clock/1 -> Switch1/2
  Constant3/1 -> Switch2/3
  Sum2/1 -> Switch2/1, Display1/1
  Switch2/1 -> To Workspace11/1
  Clock1/1 -> Switch2/2

== system MavicProComplete/Quadcopter/wind_simulator/wind_and_gust ==
  enableGusts : Inport
  period : Inport  Port=2
  amplitude : Inport  Port=3
  t : Inport  Port=4
  windDirection : Inport  Port=5
  speed : Inport  Port=6
  enableWind : Inport  Port=7
  Sum : Sum
  gust_generator : MATLAB Function  TreatAsAtomicUnit=on
  gust_to_drag : MATLAB Function  TreatAsAtomicUnit=on
  "wind_generator " : MATLAB Function  TreatAsAtomicUnit=on
  gusts : Outport
  drag : Outport  Port=2
  wires:
  period/1 -> gust_generator/1(period)
  gust_generator/1(gusts) -> Sum/1, gusts/1  "gusts"
  enableGusts/1 -> gust_generator/3(enabled)
  gust_to_drag/1(drag) -> drag/1  "drag"
  t/1 -> gust_generator/4(t), "wind_generator "/4(t)
  amplitude/1 -> gust_generator/2(amplitude)
  Sum/1 -> gust_to_drag/1(gusts)
  "wind_generator "/1(wind) -> Sum/2
  windDirection/1 -> "wind_generator "/1(direction)
  speed/1 -> "wind_generator "/2(speed)
  enableWind/1 -> "wind_generator "/3(enabled)

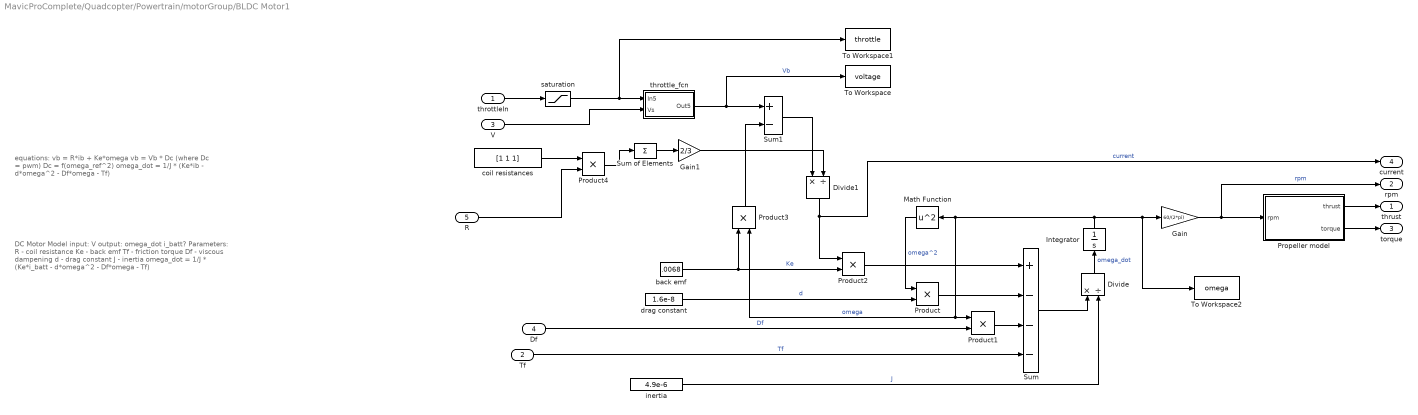
== system MavicProComplete/Quadcopter/Powertrain/motorGroup/BLDC Motor1 ==
  note: DC Motor Model
      |
      | input:
      | V
      |
      | output:
      | omega_dot
      | i_batt?
      |
      |
      | Parameters:
      | R   - coil resistance
      | Ke - back emf
      | Tf  - friction torque
      | Df  - viscous dampening
      | d   - drag constant
      | J   - inertia
      |
      | omega_dot = 1/J * (Ke*i_batt - d*omega^2 - Df*omega - Tf)
  note: equations:
      |
      | vb = R*ib + Ke*omega
      | vb = Vb * Dc  (where Dc = pwm)
      | Dc = f(omega_ref^2)
      |
      | omega_dot = 1/J * (Ke*ib - d*omega^2 - Df*omega - Tf)
  throttleIn : Inport
  Tf : Inport  Port=2
  V : Inport  Port=3
  Df : Inport  Port=4
  R : Inport  Port=5
  Divide : Product  Inputs=*/
  Divide1 : Product  Inputs=*/
  Gain : Gain  Gain=60/(2*pi)
  Gain1 : Gain  Gain=2/3
  Integrator : Integrator
  Math Function : Math  Operator=square  SaturateOnIntegerOverflow=on
  Product{,1..4} (5 alike) : Product
  "Propeller model " : MATLAB Function  TreatAsAtomicUnit=on
  Sum : Sum  Inputs=+---
  Sum of Elements : Sum  Inputs=+
  Sum1 : Sum  Inputs=+-
  To Workspace : ToWorkspace  VariableName=voltage  SaveFormat=Timeseries  SampleTime=-1
  To Workspace1 : ToWorkspace  VariableName=throttle  SaveFormat=Timeseries  SampleTime=-1
  To Workspace2 : ToWorkspace  VariableName=omega  SaveFormat=Timeseries  SampleTime=-1
  back emf : Constant  Value=.0068
  coil resistances : Constant  Value=[1 1 1]
  drag constant : Constant  Value=1.6e-8
  inertia : Constant  Value=4.9e-6
  saturation : Saturate  UpperLimit=100  LowerLimit=0
  throttle_fcn : Subsystem
  thrust : Outport
  rpm : Outport  Port=2
  torque : Outport  Port=3
  current : Outport  Port=4
  wires:
  Divide/1 -> Integrator/1  "omega_dot"
  Integrator/1 -> To Workspace2/1, Gain/1, Math Function/1, Product1/1, Product3/2  "omega"
  Gain/1 -> "Propeller model "/1(rpm), rpm/1  "rpm"
  inertia/1 -> Divide/2  "J"
  drag constant/1 -> Product/2  "d"
  Math Function/1 -> Product/1  "omega^2"
  Df/1 -> Product1/2  "Df"
  Tf/1 -> Sum/4  "Tf"
  back emf/1 -> Product3/1, Product2/2  "Ke"
  Product2/1 -> Sum/1
  Divide1/1 -> Product2/1, current/1  "current"
  V/1 -> throttle_fcn/2(Vs)
  Product3/1 -> Sum1/2
  Sum1/1 -> Divide1/1
  Gain1/1 -> Divide1/2
  "Propeller model "/1(thrust) -> thrust/1
  "Propeller model "/2(torque) -> torque/1
  Product1/1 -> Sum/3
  Product/1 -> Sum/2
  Sum/1 -> Divide/1
  coil resistances/1 -> Product4/1
  Sum of Elements/1 -> Gain1/1
  throttleIn/1 -> saturation/1
  throttle_fcn/1(Out5) -> To Workspace/1, Sum1/1  "Vb"
  saturation/1 -> To Workspace1/1, throttle_fcn/1(In5)
  R/1 -> Product4/2
  Product4/1 -> Sum of Elements/1

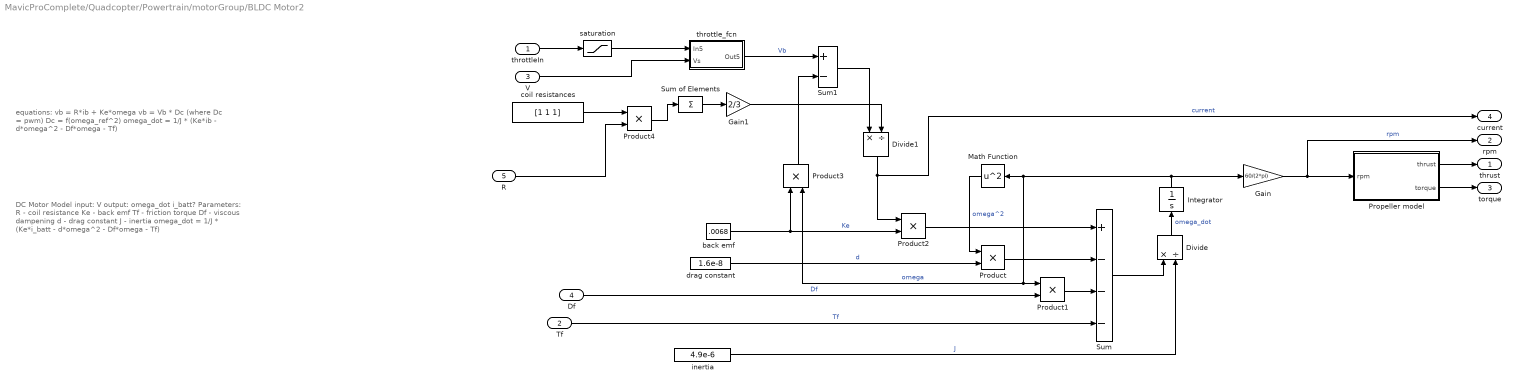
== system MavicProComplete/Quadcopter/Powertrain/motorGroup/BLDC Motor2 ==
  note: DC Motor Model
      |
      | input:
      | V
      |
      | output:
      | omega_dot
      | i_batt?
      |
      |
      | Parameters:
      | R   - coil resistance
      | Ke - back emf
      | Tf  - friction torque
      | Df  - viscous dampening
      | d   - drag constant
      | J   - inertia
      |
      | omega_dot = 1/J * (Ke*i_batt - d*omega^2 - Df*omega - Tf)
  note: equations:
      |
      | vb = R*ib + Ke*omega
      | vb = Vb * Dc  (where Dc = pwm)
      | Dc = f(omega_ref^2)
      |
      | omega_dot = 1/J * (Ke*ib - d*omega^2 - Df*omega - Tf)
  throttleIn : Inport
  Tf : Inport  Port=2
  V : Inport  Port=3
  Df : Inport  Port=4
  R : Inport  Port=5
  Divide : Product  Inputs=*/
  Divide1 : Product  Inputs=*/
  Gain : Gain  Gain=60/(2*pi)
  Gain1 : Gain  Gain=2/3
  Integrator : Integrator
  Math Function : Math  Operator=square  SaturateOnIntegerOverflow=on
  Product{,1..4} (5 alike) : Product
  "Propeller model " : MATLAB Function  TreatAsAtomicUnit=on
  Sum : Sum  Inputs=+---
  Sum of Elements : Sum  Inputs=+
  Sum1 : Sum  Inputs=+-
  back emf : Constant  Value=.0068
  coil resistances : Constant  Value=[1 1 1]
  drag constant : Constant  Value=1.6e-8
  inertia : Constant  Value=4.9e-6
  saturation : Saturate  UpperLimit=100  LowerLimit=0
  throttle_fcn : Subsystem
  thrust : Outport
  rpm : Outport  Port=2
  torque : Outport  Port=3
  current : Outport  Port=4
  wires:
  Divide/1 -> Integrator/1  "omega_dot"
  Integrator/1 -> Gain/1, Math Function/1, Product1/1, Product3/2  "omega"
  Gain/1 -> "Propeller model "/1(rpm), rpm/1  "rpm"
  inertia/1 -> Divide/2  "J"
  drag constant/1 -> Product/2  "d"
  Math Function/1 -> Product/1  "omega^2"
  Df/1 -> Product1/2  "Df"
  Tf/1 -> Sum/4  "Tf"
  back emf/1 -> Product3/1, Product2/2  "Ke"
  Product2/1 -> Sum/1
  Divide1/1 -> Product2/1, current/1  "current"
  V/1 -> throttle_fcn/2(Vs)
  Product3/1 -> Sum1/2
  Sum1/1 -> Divide1/1
  Gain1/1 -> Divide1/2
  "Propeller model "/1(thrust) -> thrust/1
  "Propeller model "/2(torque) -> torque/1
  Product1/1 -> Sum/3
  Product/1 -> Sum/2
  Sum/1 -> Divide/1
  Sum of Elements/1 -> Gain1/1
  throttleIn/1 -> saturation/1
  throttle_fcn/1(Out5) -> Sum1/1  "Vb"
  saturation/1 -> throttle_fcn/1(In5)
  coil resistances/1 -> Product4/1
  R/1 -> Product4/2
  Product4/1 -> Sum of Elements/1

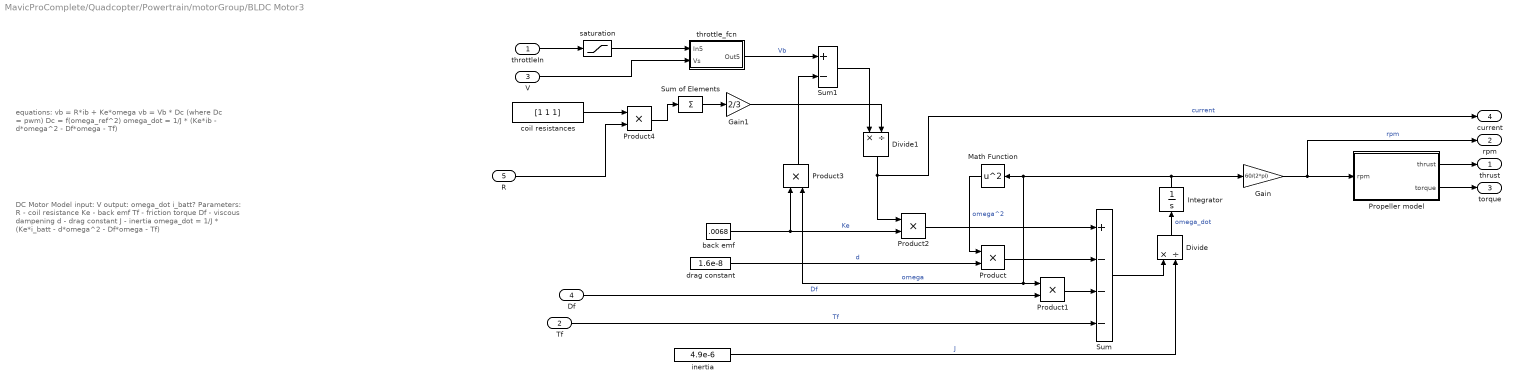
== system MavicProComplete/Quadcopter/Powertrain/motorGroup/BLDC Motor3 ==
  note: DC Motor Model
      |
      | input:
      | V
      |
      | output:
      | omega_dot
      | i_batt?
      |
      |
      | Parameters:
      | R   - coil resistance
      | Ke - back emf
      | Tf  - friction torque
      | Df  - viscous dampening
      | d   - drag constant
      | J   - inertia
      |
      | omega_dot = 1/J * (Ke*i_batt - d*omega^2 - Df*omega - Tf)
  note: equations:
      |
      | vb = R*ib + Ke*omega
      | vb = Vb * Dc  (where Dc = pwm)
      | Dc = f(omega_ref^2)
      |
      | omega_dot = 1/J * (Ke*ib - d*omega^2 - Df*omega - Tf)
  throttleIn : Inport
  Tf : Inport  Port=2
  V : Inport  Port=3
  Df : Inport  Port=4
  R : Inport  Port=5
  Divide : Product  Inputs=*/
  Divide1 : Product  Inputs=*/
  Gain : Gain  Gain=60/(2*pi)
  Gain1 : Gain  Gain=2/3
  Integrator : Integrator
  Math Function : Math  Operator=square  SaturateOnIntegerOverflow=on
  Product{,1..4} (5 alike) : Product
  "Propeller model " : MATLAB Function  TreatAsAtomicUnit=on
  Sum : Sum  Inputs=+---
  Sum of Elements : Sum  Inputs=+
  Sum1 : Sum  Inputs=+-
  back emf : Constant  Value=.0068
  coil resistances : Constant  Value=[1 1 1]
  drag constant : Constant  Value=1.6e-8
  inertia : Constant  Value=4.9e-6
  saturation : Saturate  UpperLimit=100  LowerLimit=0
  throttle_fcn : Subsystem
  thrust : Outport
  rpm : Outport  Port=2
  torque : Outport  Port=3
  current : Outport  Port=4
  wires:
  Divide/1 -> Integrator/1  "omega_dot"
  Integrator/1 -> Gain/1, Math Function/1, Product1/1, Product3/2  "omega"
  Gain/1 -> "Propeller model "/1(rpm), rpm/1  "rpm"
  inertia/1 -> Divide/2  "J"
  drag constant/1 -> Product/2  "d"
  Math Function/1 -> Product/1  "omega^2"
  Df/1 -> Product1/2  "Df"
  Tf/1 -> Sum/4  "Tf"
  back emf/1 -> Product3/1, Product2/2  "Ke"
  Product2/1 -> Sum/1
  Divide1/1 -> Product2/1, current/1  "current"
  V/1 -> throttle_fcn/2(Vs)
  Product3/1 -> Sum1/2
  Sum1/1 -> Divide1/1
  Gain1/1 -> Divide1/2
  "Propeller model "/1(thrust) -> thrust/1
  "Propeller model "/2(torque) -> torque/1
  Product1/1 -> Sum/3
  Product/1 -> Sum/2
  Sum/1 -> Divide/1
  Sum of Elements/1 -> Gain1/1
  throttleIn/1 -> saturation/1
  throttle_fcn/1(Out5) -> Sum1/1  "Vb"
  saturation/1 -> throttle_fcn/1(In5)
  coil resistances/1 -> Product4/1
  R/1 -> Product4/2
  Product4/1 -> Sum of Elements/1

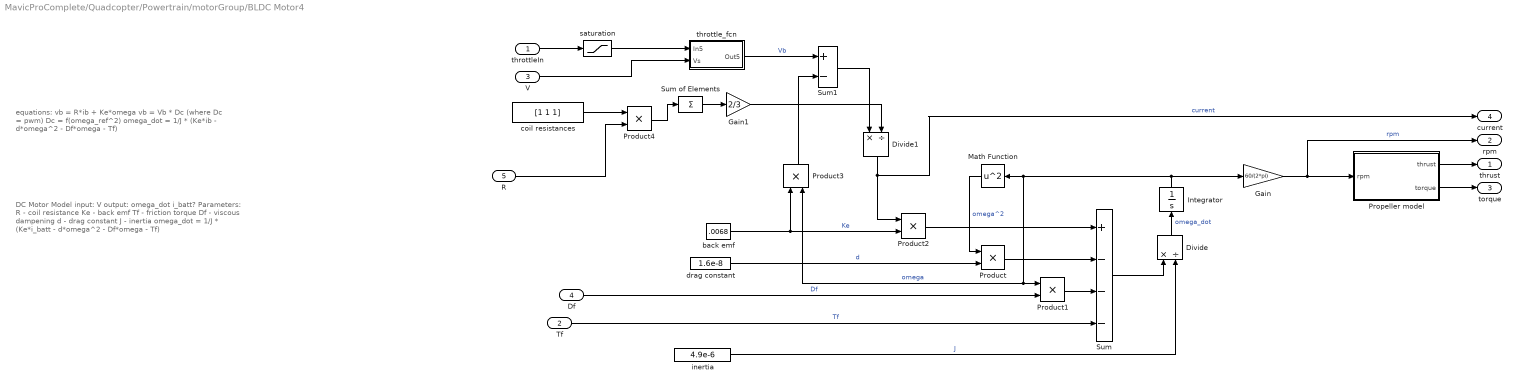
== system MavicProComplete/Quadcopter/Powertrain/motorGroup/BLDC Motor4 ==
  note: DC Motor Model
      |
      | input:
      | V
      |
      | output:
      | omega_dot
      | i_batt?
      |
      |
      | Parameters:
      | R   - coil resistance
      | Ke - back emf
      | Tf  - friction torque
      | Df  - viscous dampening
      | d   - drag constant
      | J   - inertia
      |
      | omega_dot = 1/J * (Ke*i_batt - d*omega^2 - Df*omega - Tf)
  note: equations:
      |
      | vb = R*ib + Ke*omega
      | vb = Vb * Dc  (where Dc = pwm)
      | Dc = f(omega_ref^2)
      |
      | omega_dot = 1/J * (Ke*ib - d*omega^2 - Df*omega - Tf)
  throttleIn : Inport
  Tf : Inport  Port=2
  V : Inport  Port=3
  Df : Inport  Port=4
  R : Inport  Port=5
  Divide : Product  Inputs=*/
  Divide1 : Product  Inputs=*/
  Gain : Gain  Gain=60/(2*pi)
  Gain1 : Gain  Gain=2/3
  Integrator : Integrator
  Math Function : Math  Operator=square  SaturateOnIntegerOverflow=on
  Product{,1..4} (5 alike) : Product
  "Propeller model " : MATLAB Function  TreatAsAtomicUnit=on
  Sum : Sum  Inputs=+---
  Sum of Elements : Sum  Inputs=+
  Sum1 : Sum  Inputs=+-
  back emf : Constant  Value=.0068
  coil resistances : Constant  Value=[1 1 1]
  drag constant : Constant  Value=1.6e-8
  inertia : Constant  Value=4.9e-6
  saturation : Saturate  UpperLimit=100  LowerLimit=0
  throttle_fcn : Subsystem
  thrust : Outport
  rpm : Outport  Port=2
  torque : Outport  Port=3
  current : Outport  Port=4
  wires:
  Divide/1 -> Integrator/1  "omega_dot"
  Integrator/1 -> Gain/1, Math Function/1, Product1/1, Product3/2  "omega"
  Gain/1 -> "Propeller model "/1(rpm), rpm/1  "rpm"
  inertia/1 -> Divide/2  "J"
  drag constant/1 -> Product/2  "d"
  Math Function/1 -> Product/1  "omega^2"
  Df/1 -> Product1/2  "Df"
  Tf/1 -> Sum/4  "Tf"
  back emf/1 -> Product3/1, Product2/2  "Ke"
  Product2/1 -> Sum/1
  Divide1/1 -> Product2/1, current/1  "current"
  V/1 -> throttle_fcn/2(Vs)
  Product3/1 -> Sum1/2
  Sum1/1 -> Divide1/1
  Gain1/1 -> Divide1/2
  "Propeller model "/1(thrust) -> thrust/1
  "Propeller model "/2(torque) -> torque/1
  Product1/1 -> Sum/3
  Product/1 -> Sum/2
  Sum/1 -> Divide/1
  Sum of Elements/1 -> Gain1/1
  throttleIn/1 -> saturation/1
  throttle_fcn/1(Out5) -> Sum1/1  "Vb"
  saturation/1 -> throttle_fcn/1(In5)
  coil resistances/1 -> Product4/1
  R/1 -> Product4/2
  Product4/1 -> Sum of Elements/1

== system MavicProComplete/Quadcopter/Powertrain/motorGroup/Subsystem ==
  throttle : Inport
  voltage : Inport  Port=2
  Df : Inport  Port=3
  Constant3 : Constant  Value=.1
  Constant4 : Constant  Value=.0000001
  Level-2 MATLAB S-Function : M-S-Function  FunctionName=motorUKF_Sfcn  Parameters=motorParams
      mask Display:
      | port_label('input', 1, 'voltage');
      | port_label('input', 2, 'friction');
      | port_label('output', 1, 'current');
      | port_label('output', 2, 'rpm_hat');
      | disp("Motor UKF");
  MATLAB Function : MATLAB Function  TreatAsAtomicUnit=on
  MATLAB Function1 : MATLAB Function  TreatAsAtomicUnit=on
  Median Filter : dspstat3/Median Filter  WindowLength=100  SimulateUsing=Interpreted execution
      settings: SourceProductName=DSP System Toolbox  SourceProductBaseCode=DS
  Scope5 : Scope
  saturation : Saturate  UpperLimit=100  LowerLimit=0
  throttle_fcn : Subsystem
  estimated_rpm : Outport
  estimated_current : Outport  Port=2
  wires:
  Constant4/1 -> MATLAB Function1/2(sigma)
  throttle/1 -> saturation/1
  MATLAB Function/1(y) -> Scope5/1, Level-2 MATLAB S-Function/1
  throttle_fcn/1(Out5) -> MATLAB Function/1(mu)  "Vb"
  Level-2 MATLAB S-Function/2 -> estimated_rpm/1  "estimated_rpm"
  Median Filter/1 -> estimated_current/1  "estimated_current"
  MATLAB Function1/1(y) -> Level-2 MATLAB S-Function/2
  Level-2 MATLAB S-Function/1 -> Median Filter/1  "estimated_current"
  voltage/1 -> throttle_fcn/2(Vs)
  Df/1 -> MATLAB Function1/1(mu)
  saturation/1 -> throttle_fcn/1(In5)
  Constant3/1 -> MATLAB Function/2(sigma)

== system MavicProComplete/Quadcopter/Powertrain/motorGroup/BLDC Motor1/throttle_fcn ==
  note: Output equals linearly scaled RPM
      | for given throttle input if throttle input >=Throttle Cuttoff (minThr)
      | else output is zero.
  In5 : Inport
  Vs : Inport  Port=2
  Gain : Gain  Gain=.01
  Minimum Throttle Cutoff : simulink/Logic and Bit Operations/Compare To Constant  relop=>=  const=5  OutDataTypeStr=uint8
  Product : Product
  Product2 : Product  OutDataTypeStr=double
  Out5 : Outport
  wires:
  Minimum Throttle Cutoff/1 -> Product/2
  Product/1 -> Out5/1
  In5/1 -> Gain/1, Minimum Throttle Cutoff/1
  Gain/1 -> Product2/2
  Product2/1 -> Product/1
  Vs/1 -> Product2/1

== system MavicProComplete/Quadcopter/Powertrain/motorGroup/BLDC Motor2/throttle_fcn ==
  note: Output equals linearly scaled RPM
      | for given throttle input if throttle input >=Throttle Cuttoff (minThr)
      | else output is zero.
  In5 : Inport
  Vs : Inport  Port=2
  Gain : Gain  Gain=.01
  Minimum Throttle Cutoff : simulink/Logic and Bit Operations/Compare To Constant  relop=>=  const=5  OutDataTypeStr=uint8
  Product : Product
  Product2 : Product  OutDataTypeStr=double
  Out5 : Outport
  wires:
  Minimum Throttle Cutoff/1 -> Product/2
  Product/1 -> Out5/1
  In5/1 -> Gain/1, Minimum Throttle Cutoff/1
  Gain/1 -> Product2/2
  Product2/1 -> Product/1
  Vs/1 -> Product2/1
